simulink model "MPC_3Phase_Inverter"  (R2021a)
settings: Solver=ode45  StartTime=0  StopTime=0.5  MaxStep=3.3E-5  RelTol=1e-3  EnableMultiTasking=on
values from neighbouring files (symbols this model uses):
  Cfilter = 40e-6    (= 4e-05)    [init_inverter.m]
  Lfilter = 2.4e-3    (= 0.0024)    [init_inverter.m]
  Res = 50    [init_inverter.m]
  Ts = 1e-5    (= 1e-05)    [init_inverter.m]
  Vdc = 400    [init_inverter.m]
  Vref = 188    [init_inverter.m]
undefined symbols (not defined in the file or in its folder): i
libraries: simulink x7, spsIGBTDiodeLib x6, spsGroundLib x4, spsThreePhaseSeriesRLCBranchLib x3, spsCurrentMeasurementLib x3, spsThreePhaseVIMeasurementLib x2, spspowerguiLib x2, spsDCVoltageSourceLib x1
settings Model: Creator=ENG.Ihab  LastModifiedBy=Kuhan
settings SolverCC: AlgebraicLoopSolver=TrustRegion  AutoInsertRateTranBlk=on
settings DataIOCC: LimitDataPoints=on  SaveFormat=Array  SignalLoggingSaveFormat=ModelDataLogs  ReturnWorkspaceOutputs=off
settings OptimizationCC: ExpressionDepthLimit=2147483647  LifeSpan=inf
settings DebuggingCC: AlgebraicLoopMsg=none  UnderspecifiedInitializationDetection=Classic  MergeDetectMultiDrivingBlocksExec=none  FcnCallInpInsideContextMsg=warning  UnconnectedInputMsg=none  UnconnectedOutputMsg=none  UnconnectedLineMsg=none  StateNameClashWarn=warning  SFUnexpectedBacktrackingDiag=warning  SFNoUnconditionalDefaultTransitionDiag=warning  SFExecutionAtInitializationDiag=none  SFMachineParentedDataDiag=warning  ArithmeticOperatorsInVariantConditions=warning
settings HardwareCC: ProdBitPerPointer=32  ProdBitPerSizeT=32  ProdBitPerPtrDiffT=32  ProdLargestAtomicFloat=None  ProdIntDivRoundTo=Undefined  ProdEndianess=Unspecified  ProdWordSize=32  ProdHWDeviceType=32-bit Generic
settings ModelReferenceCC: PropagateSignalLabelsOutOfModel=off
settings SFSimCC: SimUseLocalCustomCode=off  SimParseCustomCode=off  CustomCodeUndefinedFunction=UseInterfaceOnly
settings RTWCC: RTWUseLocalCustomCode=off
settings CodeAppCC: StateflowObjectComments=on
settings GRTTargetCC: TargetLangStandard=C89/C90 (ANSI)  CombineOutputUpdateFcns=off  GRTInterface=on
settings ConfigComp: CovMetricSettings=dw  CovSaveCumulativeToWorkspaceVar=on  CovSaveSingleToWorkspaceVar=on  CovExternalEMLEnable=off

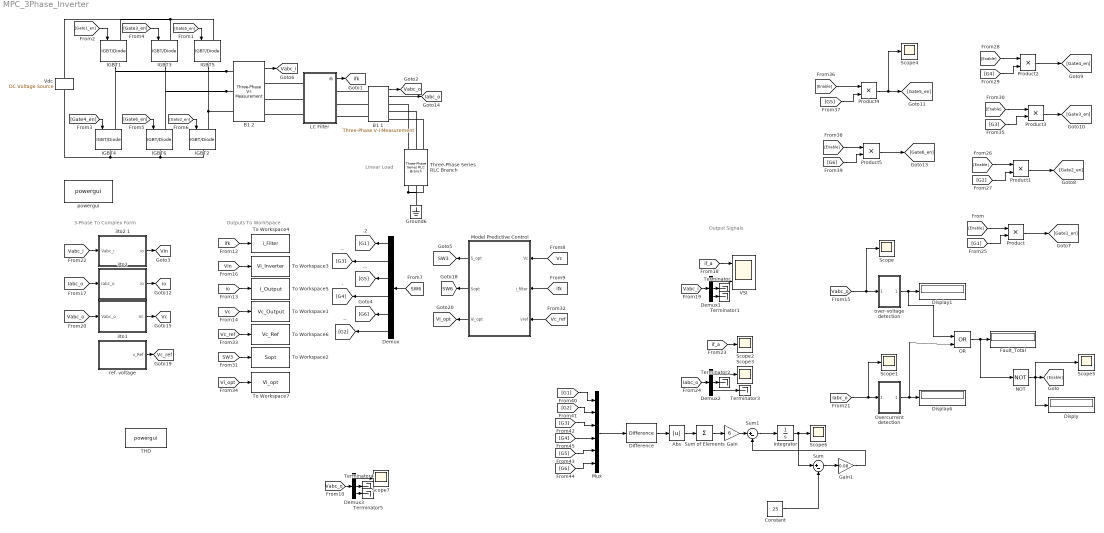
== system MPC_3Phase_Inverter ==
  note: Linear Load
  note: Outputs To WorkSpace
  note: Output Signals
  note: 3-Phase To Complex Form
  3to1 : Subsystem
  "3to2 " : Subsystem
  3to2 1 : Subsystem
  Abs : Abs
  B1 1 : spsThreePhaseVIMeasurementLib/Three-Phase V-I Measurement  VoltageMeasurement=phase-to-ground  SetLabelV=off  LabelV=Vabc  Vpu=off  VpuLL=off  CurrentMeasurement=yes  SetLabelI=off  LabelI=Iabc  Ipu=off  Pbase=100e6  Vbase=500e3  OutputType=Complex  PhasorSimulation=off  PSBequivalent=0
  B1 2 : spsThreePhaseVIMeasurementLib/Three-Phase V-I Measurement  VoltageMeasurement=phase-to-ground  SetLabelV=off  LabelV=Vabc  Vpu=off  VpuLL=off  CurrentMeasurement=no  SetLabelI=off  LabelI=Iabc  Ipu=off  Pbase=100e6  Vbase=500e3  OutputType=Complex  PhasorSimulation=off  PSBequivalent=0
  Constant : Constant  Value=25
  Demux : Demux  Outputs=6
  Demux1 : Demux  Outputs=3
  Demux2 : Demux  Outputs=3
  Demux3 : Demux  Outputs=3
  Difference : simulink/Discrete/Difference  ICPrevInput=0.0  OutMin=[]  OutMax=[]  OutDataType=fixdt(1, 16)  OutScaling=2^-10  DoSatur=off
  Display1 : Display
  Display6 : Display
  Disply : Display
  Fault_Total : Display
  Gain : Gain  Gain=6
  Gain1 : Gain  Gain=0.08
  Ground6 : spsGroundLib/Ground  LConnTagsString=a
  IGBT{1..6} (6 alike) : spsIGBTDiodeLib/IGBT//Diode  Ron=1e-3  Rs=1e5  Cs=inf  Measurements=off
  Integrator : Integrator  InitialCondition=25
  LC Filter : Subsystem
  "Model Predictive Control " : MATLAB Function  TreatAsAtomicUnit=on  mask{Ts=Ts, Cfilter=Cfilter, Lfilter=Lfilter, Vdc=Vdc}
      mask prompts: Ts "Sampling Time"; Cfilter "Filter Capacitor"; Lfilter "Filter Inductance"; Vdc "Input DC Voltage"
  Mux : Mux  Inputs=6
  NOT : Logic  Operator=NOT  IconShape=distinctive  AllPortsSameDT=off  OutDataTypeStr=boolean
  OR : Logic  Operator=OR  IconShape=distinctive  AllPortsSameDT=off  OutDataTypeStr=boolean
  Overcurrent detection : Subsystem
  Product{,1..5} (6 alike) : Product
  Scope{,1..7} (8 alike) : Scope
  Sum : Sum  Inputs=|+-
  Sum of Elements : Sum  Inputs=+
  Sum1 : Sum  Inputs=|+-
  THD : spspowerguiLib/powergui  Priority=1  SimulationMode=Continuous  SampleTime=50e-6  frequency=60  Iterations=50  frequencyindice=60  Pbase=100e6  ErrMax=1e-4  UnitsV=kV  UnitsW=MW  buscounter=0  FunctionMessages=off  echomessages=off  EnableUseOfTLC=off  CurrentSourceSwitches=off  DisableSnubberDevices=off  DisableRonSwitches=off  DisableVfSwitches=off  DisplayEquations=off  AutomaticDiscreteSolvers=off  SolverType=Tustin/Backward Euler (TBE)  Interpol=off  ExternalGateDelay=off  methode=off  Ts=100  x0status=blocks  SPID=on  SwTol=0  HookPort=off  NonlinearTolerance=1e-4  nMaxIteration=100  ContinueOnMaxIteration=off  RestoreLinks=warning  ResistiveCurrentMeasurement=off  Frange=[0:2:500]  Ylog=off  Xlog=on  ShowGrid=off  save=off  variable=ZData  structure=0  ZoomFFT=off  StartTime=0.0  cycles=1  DisplayStyle=1  fundamental=60  FreqAxis=off  MaxFrequency=1000  frequencyindicesteady=1  RmsSteady=1  display=off
  Terminator{,1..5} (6 alike) : Terminator
  Three-Phase Series RLC Branch : spsThreePhaseSeriesRLCBranchLib/Three-Phase Series RLC Branch  LConnTagsString=A|B|C  RConnTagsString=A|B|C  BranchType=R  Resistance=Res  Inductance=0.01  Capacitance=40e-6  Measurements=None
  To Workspace1 : ToWorkspace  VariableName=Vc_Output  SampleTime=-1
  To Workspace2 : ToWorkspace  VariableName=Sopt  SaveFormat=Structure With Time  SampleTime=-1
      settings: Save2DSignal=2-D array (concatenate along first dimension)
  To Workspace3 : ToWorkspace  VariableName=Vi_Inverter  SampleTime=-1
  To Workspace4 : ToWorkspace  VariableName=i_Filter  SampleTime=-1
  To Workspace5 : ToWorkspace  VariableName=i_Output  SampleTime=-1
  To Workspace6 : ToWorkspace  VariableName=Vc_Ref  SampleTime=-1
  To Workspace7 : ToWorkspace  VariableName=Vi_opt  SampleTime=-1
      settings: Save2DSignal=2-D array (concatenate along first dimension)
  VSI : Scope  NumInputPorts=2
  Vdc : spsDCVoltageSourceLib/DC Voltage Source  Description=source block  Amplitude=Vdc  Measurements=None
      settings: AttributesFormatString=\n
  over-voltage detection : Subsystem
  powergui : spspowerguiLib/powergui  SimulationMode=Discrete  SampleTime=Ts  frequency=60  Iterations=50  frequencyindice=0  Pbase=100e6  ErrMax=1e-4  UnitsV=kV  UnitsW=MW  buscounter=0  FunctionMessages=off  echomessages=off  EnableUseOfTLC=off  CurrentSourceSwitches=off  DisableSnubberDevices=off  DisableRonSwitches=off  DisableVfSwitches=off  DisplayEquations=off  AutomaticDiscreteSolvers=off  SolverType=Tustin/Backward Euler (TBE)  Interpol=off  ExternalGateDelay=off  methode=off  Ts=100  x0status=blocks  SPID=off  SwTol=0  HookPort=off  NonlinearTolerance=1e-4  nMaxIteration=100  ContinueOnMaxIteration=off  RestoreLinks=warning  ResistiveCurrentMeasurement=off  Frange=[0:2:500]  Ylog=off  Xlog=on  ShowGrid=off  save=off  variable=ZData  structure=Outputs  ZoomFFT=off  StartTime=0.07  cycles=2  DisplayStyle=1  fundamental=50  FreqAxis=on  MaxFrequency=2000  frequencyindicesteady=1  RmsSteady=2  display=off
  ref. voltage : Subsystem
  tag scope: Iabc_o=global, SW3=global, SW6=global, Vabc_i=global, Vabc_o=global, Vc=global, Vc_ref=global, Vi_opt=global, Vin=global, ifk=global, io=global
  wires:
  LC Filter/1(ifk) -> [ifk]
  [Gate4_en] -> IGBT4/1
  [Gate3_en] -> IGBT3/1
  [Gate6_en] -> IGBT6/1
  [Gate2_en] -> IGBT2/1
  [Gate5_en] -> IGBT5/1
  [Gate1_en] -> IGBT1/1
  Demux/1 -> [G1]
  Demux/2 -> [G3]
  Demux/3 -> [G5]
  Demux/4 -> [G4]
  Demux/5 -> [G6]
  Demux/6 -> [G2]
  "Model Predictive Control "/1(S_opt) -> [SW3]
  [SW6] -> Demux/1
  [Vc] -> "Model Predictive Control "/1(Vc)
  [ifk] -> "Model Predictive Control "/2(i_filter)
  [ifk] -> To Workspace4/1
  [Vin] -> To Workspace3/1
  "3to2 "/1(io) -> [io]
  3to1/1(Vc) -> [Vc]
  [io] -> To Workspace5/1
  [Vc] -> To Workspace1/1
  [SW3] -> To Workspace2/1
  "Model Predictive Control "/2(Sopt) -> [SW6]
  [Vc_ref] -> "Model Predictive Control "/3(vref)
  [Vc_ref] -> To Workspace6/1
  ref. voltage/1(v_Ref) -> [Vc_ref]
  "Model Predictive Control "/3(Vi_opt) -> [Vi_opt]
  [Vi_opt] -> To Workspace7/1
  B1 1/2 -> [Iabc_o]
  [Iabc_o] -> "3to2 "/1("Iabc_o ")
  B1 1/1 -> [Vabc_o]
  [Vabc_o] -> 3to1/1("Vabc_o ")
  B1 2/1 -> [Vabc_i]
  [Vabc_i] -> 3to2 1/1("Vabc_i ")
  3to2 1/1(io) -> [Vin]
  [if_a] -> VSI/1
  Demux1/2 -> Terminator/1
  [Vabc_i] -> Demux1/1
  Demux1/1 -> VSI/2
  Demux1/3 -> Terminator1/1
  [Vabc_o] -> over-voltage detection/1(In1), Scope/1
  [if_a] -> Scope2/1
  Demux2/3 -> Terminator3/1
  [Iabc_o] -> Demux2/1
  Demux2/2 -> Terminator2/1
  Demux2/1 -> Scope3/1
  [Iabc_o] -> Scope1/1, Overcurrent detection/1(In1)
  Overcurrent detection/1(Out1) -> OR/2, Display6/1
  over-voltage detection/1(Out1) -> OR/1, Display1/1
  OR/1 -> NOT/1, Fault_Total/1
  [Enable] -> Product/1
  [G1] -> Product/2
  Product/1 -> [Gate1_en]
  [Enable] -> Product1/1
  [G2] -> Product1/2
  Product1/1 -> [Gate2_en]
  [G4] -> Product2/2
  Product2/1 -> [Gate4_en]
  [Enable] -> Product2/1
  [G3] -> Product3/2
  Product3/1 -> [Gate3_en]
  [Enable] -> Product3/1
  [G5] -> Product4/2
  [Enable] -> Product4/1
  Product4/1 -> Scope4/1, [Gate5_en]
  [G6] -> Product5/2
  [Enable] -> Product5/1
  Product5/1 -> [Gate6_en]
  NOT/1 -> Scope5/1, Disply/1, [Enable]
  Difference/1 -> Abs/1
  [G1] -> Mux/1
  [G2] -> Mux/2
  [G4] -> Mux/4
  [G3] -> Mux/3
  [G5] -> Mux/5
  [G6] -> Mux/6
  Mux/1 -> Difference/1
  Abs/1 -> Sum of Elements/1
  Sum of Elements/1 -> Gain/1
  Integrator/1 -> Sum/1, Scope6/1
  Constant/1 -> Sum/2
  Sum/1 -> Gain1/1
  Gain/1 -> Sum1/1
  Sum1/1 -> Integrator/1
  Gain1/1 -> Sum1/2
  Demux3/3 -> Terminator5/1
  Demux3/1 -> Scope7/1
  [Vabc_o] -> Demux3/1
  Demux3/2 -> Terminator4/1
  connections:
  IGBT2/RConn1 -- IGBT6/RConn1 -- Vdc/LConn1 -- IGBT4/RConn1
  IGBT1/LConn1 -- Vdc/RConn1 -- IGBT3/LConn1 -- IGBT5/LConn1
  B1 2/LConn1 -- IGBT4/LConn1 -- IGBT1/RConn1
  IGBT5/RConn1 -- B1 2/LConn3 -- IGBT2/LConn1
  B1 2/LConn2 -- IGBT6/LConn1 -- IGBT3/RConn1
  B1 1/LConn3 -- LC Filter/RConn3
  B1 1/LConn2 -- LC Filter/RConn2
  B1 1/LConn1 -- LC Filter/RConn1
  Three-Phase Series RLC Branch/RConn1 -- B1 1/RConn1
  Three-Phase Series RLC Branch/RConn2 -- B1 1/RConn2
  Three-Phase Series RLC Branch/RConn3 -- B1 1/RConn3
  LC Filter/LConn3 -- B1 2/RConn3
  LC Filter/LConn2 -- B1 2/RConn2
  LC Filter/LConn1 -- B1 2/RConn1
  Three-Phase Series RLC Branch/LConn1 -- Three-Phase Series RLC Branch/LConn2 -- Three-Phase Series RLC Branch/LConn3 -- Ground6/LConn1

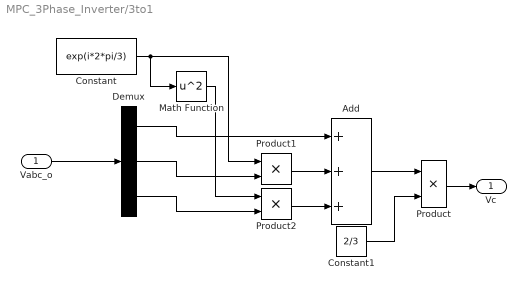
== system MPC_3Phase_Inverter/3to1 ==
  "Vabc_o " : Inport
  Add : Sum  Inputs=+++
  Constant : Constant  Value=exp(i*2*pi/3)
  Constant1 : Constant  Value=2/3
  Demux : Demux  Outputs=3
  Math Function : Math  Operator=square  SignedPower=on  SaturateOnIntegerOverflow=on
  Product : Product  RndMeth=Zero
  Product1 : Product  RndMeth=Zero
  Product2 : Product  RndMeth=Zero
  Vc : Outport  VectorParamsAs1DForOutWhenUnconnected=off
  wires:
  Demux/2 -> Product1/2
  Demux/3 -> Product2/2
  Product2/1 -> Add/3
  Constant1/1 -> Product/2
  Math Function/1 -> Product2/1
  Product/1 -> Vc/1
  Add/1 -> Product/1
  "Vabc_o "/1 -> Demux/1
  Constant/1 -> Product1/1, Math Function/1
  Demux/1 -> Add/1
  Product1/1 -> Add/2

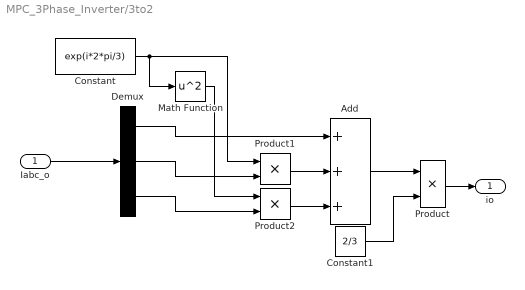
== system MPC_3Phase_Inverter/3to2  ==
  "Iabc_o " : Inport
  Add : Sum  Inputs=+++
  Constant : Constant  Value=exp(i*2*pi/3)
  Constant1 : Constant  Value=2/3
  Demux : Demux  Outputs=3
  Math Function : Math  Operator=square  SignedPower=on  SaturateOnIntegerOverflow=on
  Product : Product  RndMeth=Zero
  Product1 : Product  RndMeth=Zero
  Product2 : Product  RndMeth=Zero
  io : Outport  VectorParamsAs1DForOutWhenUnconnected=off
  wires:
  Add/1 -> Product/1
  Demux/1 -> Add/1
  Constant1/1 -> Product/2
  Product1/1 -> Add/2
  Constant/1 -> Product1/1, Math Function/1
  Demux/2 -> Product1/2
  Math Function/1 -> Product2/1
  Demux/3 -> Product2/2
  Product2/1 -> Add/3
  Product/1 -> io/1
  "Iabc_o "/1 -> Demux/1

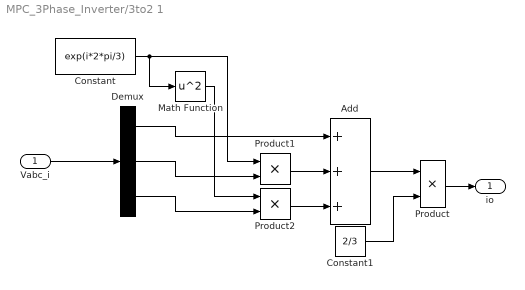
== system MPC_3Phase_Inverter/3to2 1 ==
  "Vabc_i " : Inport
  Add : Sum  Inputs=+++
  Constant : Constant  Value=exp(i*2*pi/3)
  Constant1 : Constant  Value=2/3
  Demux : Demux  Outputs=3
  Math Function : Math  Operator=square  SignedPower=on  SaturateOnIntegerOverflow=on
  Product : Product  RndMeth=Zero
  Product1 : Product  RndMeth=Zero
  Product2 : Product  RndMeth=Zero
  io : Outport  VectorParamsAs1DForOutWhenUnconnected=off
  wires:
  Add/1 -> Product/1
  Demux/1 -> Add/1
  Constant1/1 -> Product/2
  Product1/1 -> Add/2
  Constant/1 -> Product1/1, Math Function/1
  Demux/2 -> Product1/2
  Math Function/1 -> Product2/1
  Demux/3 -> Product2/2
  Product2/1 -> Add/3
  Product/1 -> io/1
  "Vabc_i "/1 -> Demux/1

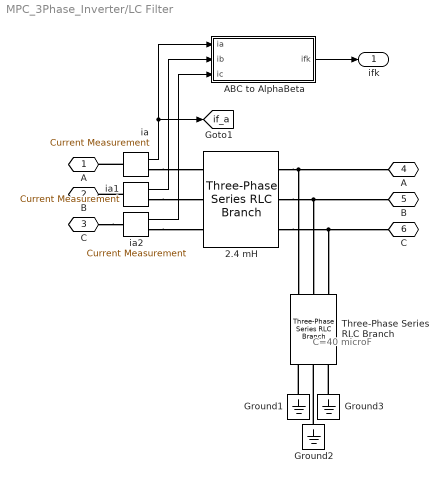
== system MPC_3Phase_Inverter/LC Filter ==
  note: C=40 microF
  "2.4 mH " : spsThreePhaseSeriesRLCBranchLib/Three-Phase Series RLC Branch  LConnTagsString=A|B|C  RConnTagsString=A|B|C  BranchType=L  Resistance=1.0  Inductance=Lfilter  Capacitance=1.0  Measurements=None
  "ABC to AlphaBeta " : Subsystem
  Ground1 : spsGroundLib/Ground  LConnTagsString=a
  Ground2 : spsGroundLib/Ground  LConnTagsString=a
  Ground3 : spsGroundLib/Ground  LConnTagsString=a
  Three-Phase Series RLC Branch : spsThreePhaseSeriesRLCBranchLib/Three-Phase Series RLC Branch  LConnTagsString=A|B|C  RConnTagsString=A|B|C  BranchType=C  Resistance=1  Inductance=1e-3  Capacitance=Cfilter  Measurements=None
  ia : spsCurrentMeasurementLib/Current Measurement  PhasorSimulation=off  OutputType=Complex  PSBequivalent=0
  ia1 : spsCurrentMeasurementLib/Current Measurement  PhasorSimulation=off  OutputType=Complex  PSBequivalent=0
  ia2 : spsCurrentMeasurementLib/Current Measurement  PhasorSimulation=off  OutputType=Complex  PSBequivalent=0
  A : PMIOPort  Side=Left
  B : PMIOPort  Port=2  Side=Left
  C : PMIOPort  Port=3  Side=Left
  "A " : PMIOPort  Port=4  Side=Right
  "B " : PMIOPort  Port=5  Side=Right
  "C " : PMIOPort  Port=6  Side=Right
  ifk : Outport  VectorParamsAs1DForOutWhenUnconnected=off
  tag scope: if_a=global
  wires:
  ia/1 -> [if_a], "ABC to AlphaBeta "/1(ia)
  ia1/1 -> "ABC to AlphaBeta "/2(ib)
  ia2/1 -> "ABC to AlphaBeta "/3(ic)
  "ABC to AlphaBeta "/1(ifk) -> ifk/1
  connections:
  "2.4 mH "/RConn1 -- Three-Phase Series RLC Branch/RConn1 -- "A "/RConn1
  "2.4 mH "/RConn2 -- Three-Phase Series RLC Branch/RConn2 -- "B "/RConn1
  "2.4 mH "/RConn3 -- Three-Phase Series RLC Branch/RConn3 -- "C "/RConn1
  ia/LConn1 -- A/RConn1
  ia/RConn1 -- "2.4 mH "/LConn1
  ia1/LConn1 -- B/RConn1
  C/RConn1 -- ia2/LConn1
  ia1/RConn1 -- "2.4 mH "/LConn2
  ia2/RConn1 -- "2.4 mH "/LConn3
  Ground1/LConn1 -- Three-Phase Series RLC Branch/LConn1
  Ground2/LConn1 -- Three-Phase Series RLC Branch/LConn2
  Ground3/LConn1 -- Three-Phase Series RLC Branch/LConn3

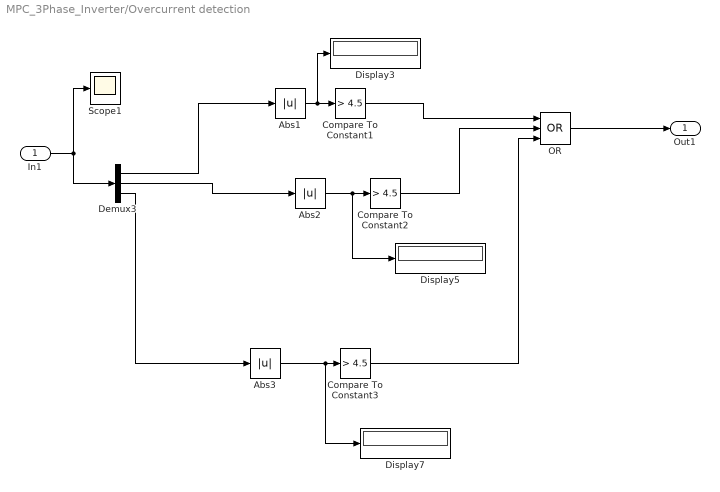
== system MPC_3Phase_Inverter/Overcurrent detection ==
  In1 : Inport
  Abs1 : Abs
  Abs2 : Abs
  Abs3 : Abs
  Compare To Constant1 : simulink/Logic and Bit Operations/Compare To Constant  relop=>  const=4.5  OutDataTypeStr=boolean
  Compare To Constant2 : simulink/Logic and Bit Operations/Compare To Constant  relop=>  const=4.5  OutDataTypeStr=boolean
  Compare To Constant3 : simulink/Logic and Bit Operations/Compare To Constant  relop=>  const=4.5  OutDataTypeStr=boolean
  Demux3 : Demux  Outputs=3
  Display3 : Display
  Display5 : Display
  Display7 : Display
  OR : Logic  Operator=OR  Inputs=3  IconShape=distinctive  AllPortsSameDT=off  OutDataTypeStr=boolean
  Scope1 : Scope
  Out1 : Outport
  wires:
  Abs3/1 -> Display7/1, Compare To Constant3/1
  Demux3/1 -> Abs1/1
  Compare To Constant2/1 -> OR/2
  In1/1 -> Scope1/1, Demux3/1
  Abs1/1 -> Display3/1, Compare To Constant1/1
  Demux3/2 -> Abs2/1
  Compare To Constant3/1 -> OR/3
  Abs2/1 -> Display5/1, Compare To Constant2/1
  Compare To Constant1/1 -> OR/1
  Demux3/3 -> Abs3/1
  OR/1 -> Out1/1

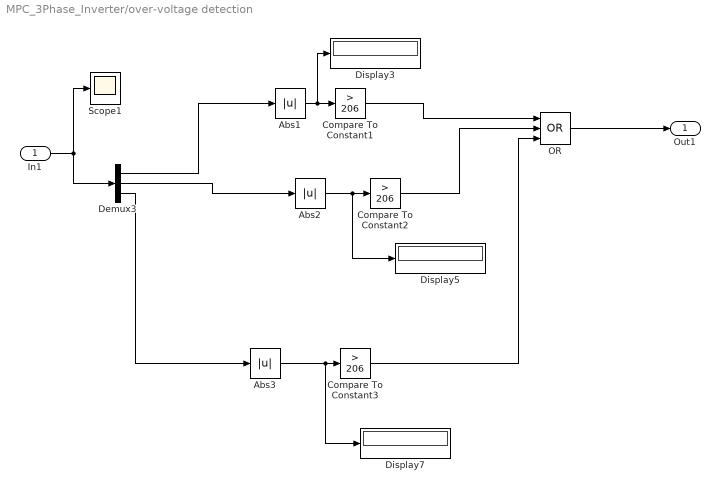
== system MPC_3Phase_Inverter/over-voltage detection ==
  In1 : Inport
  Abs1 : Abs
  Abs2 : Abs
  Abs3 : Abs
  Compare To Constant1 : simulink/Logic and Bit Operations/Compare To Constant  relop=>  const=206  OutDataTypeStr=boolean
  Compare To Constant2 : simulink/Logic and Bit Operations/Compare To Constant  relop=>  const=206  OutDataTypeStr=boolean
  Compare To Constant3 : simulink/Logic and Bit Operations/Compare To Constant  relop=>  const=206  OutDataTypeStr=boolean
  Demux3 : Demux  Outputs=3
  Display3 : Display
  Display5 : Display
  Display7 : Display
  OR : Logic  Operator=OR  Inputs=3  IconShape=distinctive  AllPortsSameDT=off  OutDataTypeStr=boolean
  Scope1 : Scope
  Out1 : Outport
  wires:
  Abs3/1 -> Display7/1, Compare To Constant3/1
  Demux3/1 -> Abs1/1
  Compare To Constant2/1 -> OR/2
  In1/1 -> Scope1/1, Demux3/1
  Abs1/1 -> Display3/1, Compare To Constant1/1
  Demux3/2 -> Abs2/1
  Compare To Constant3/1 -> OR/3
  Abs2/1 -> Display5/1, Compare To Constant2/1
  Compare To Constant1/1 -> OR/1
  Demux3/3 -> Abs3/1
  OR/1 -> Out1/1

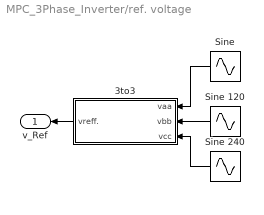
== system MPC_3Phase_Inverter/ref. voltage ==
  3to3 : Subsystem
  Sine : Sin  Amplitude=Vref  Frequency=100*pi  SampleTime=Ts
  Sine 120 : Sin  Amplitude=Vref  Frequency=100*pi  Phase=(2*pi)/3  SampleTime=Ts
  Sine 240 : Sin  Amplitude=Vref  Frequency=100*pi  Phase=(4*pi)/3  SampleTime=Ts
  v_Ref : Outport  VectorParamsAs1DForOutWhenUnconnected=off
  wires:
  Sine/1 -> 3to3/1(vaa)
  Sine 120/1 -> 3to3/2(vbb)
  Sine 240/1 -> 3to3/3(vcc)
  3to3/1(vreff.) -> v_Ref/1

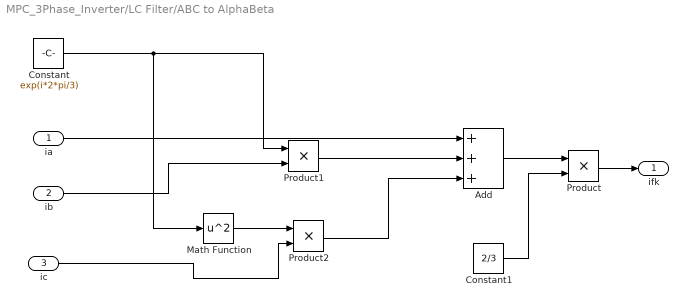
== system MPC_3Phase_Inverter/LC Filter/ABC to AlphaBeta  ==
  ia : Inport
  ib : Inport  Port=2
  ic : Inport  Port=3
  Add : Sum  Inputs=+++
  Constant : Constant  Value=exp(i*2*pi/3)
  Constant1 : Constant  Value=2/3
  Math Function : Math  Operator=square  SignedPower=on  SaturateOnIntegerOverflow=on
  Product : Product  RndMeth=Zero
  Product1 : Product  RndMeth=Zero
  Product2 : Product  RndMeth=Zero
  ifk : Outport  VectorParamsAs1DForOutWhenUnconnected=off
  wires:
  Add/1 -> Product/1
  ia/1 -> Add/1
  Constant1/1 -> Product/2
  Product1/1 -> Add/2
  Constant/1 -> Product1/1, Math Function/1
  ib/1 -> Product1/2
  Math Function/1 -> Product2/1
  ic/1 -> Product2/2
  Product2/1 -> Add/3
  Product/1 -> ifk/1

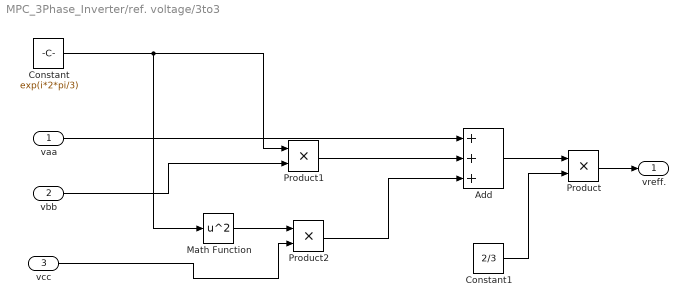
== system MPC_3Phase_Inverter/ref. voltage/3to3 ==
  vaa : Inport
  vbb : Inport  Port=2
  vcc : Inport  Port=3
  Add : Sum  Inputs=+++
  Constant : Constant  Value=exp(i*2*pi/3)
  Constant1 : Constant  Value=2/3
  Math Function : Math  Operator=square  SignedPower=on  SaturateOnIntegerOverflow=on
  Product : Product  RndMeth=Zero
  Product1 : Product  RndMeth=Zero
  Product2 : Product  RndMeth=Zero
  vreff. : Outport  VectorParamsAs1DForOutWhenUnconnected=off
  wires:
  Add/1 -> Product/1
  vaa/1 -> Add/1
  Constant1/1 -> Product/2
  Product1/1 -> Add/2
  Constant/1 -> Product1/1, Math Function/1
  vbb/1 -> Product1/2
  Math Function/1 -> Product2/1
  vcc/1 -> Product2/2
  Product2/1 -> Add/3
  Product/1 -> vreff./1

== matlab function MPC_3Phase_Inverter/Model Predictive Control  ==
  settings: sampleTime=33*1e-6
  data: S_opt output; Sopt output; Vc input; i_filter input; vref input; Vi_opt output; Vdc parameter double size=1; Ts parameter size=1; Cfilter parameter size=1; Lfilter parameter size=1
function [S_opt, Sopt, Vi_opt] = MPC(Vc,i_filter,vref,Vdc,Ts,Cfilter,Lfilter)

    % In order to call "cont2dis" function
    coder.extrinsic('cont2dis');
    persistent Aq Bq Bdq Vc1 Vc_old if_old x_opt g 

    % Initialize variables and get the parameters of the Discrete model based on Ts
    if isempty(x_opt), x_opt = 1; end
    if isempty(Vc1), Vc1 = 0 + 1j*0; end
    if isempty(Vc_old), Vc_old = 0 + 1j*0; end
    if isempty(if_old), if_old = 0 + 1j*0; end
    
    if isempty(Aq) && isempty(Bq) && isempty(Bdq)
        Aq = zeros(2);     Bq = zeros(2,1);     Bdq = zeros(2,1);
        % Call "cont2dis" function
        [Aq, Bq, Bdq] = cont2dis(Ts,Lfilter,Cfilter); 
    end
    
    % Intialize the cost function
    g_opt = inf;
    
    % To generate the switching states matrix
    states = [1 0 0;
              1 1 0
              0 1 0
              0 1 1
              0 0 1
              1 0 1
              1 1 1];
    a = exp(1j*(2*pi/3));
    
    % Read current measurements at sampling instant k
    ifk = i_filter;
    Vck = Vc;
    % Equation of io(k-1) = if(k-1)-(c/Ts)(vc(k)-vc(k-1)).
    io = if_old - (Cfilter/Ts)*(Vck - Vc_old); 
    
    % Store the measured current for the next iteration
    if_old = ifk;
    Vc_old = Vck;
    % FOR loop to find the best switch in the next instant and its corresponding V(i)
    for k = 1:7
        s = states(k,:);
        sw = (2/3)*(s(1)+a*s(2)+a^2*s(3));
        Vi = Vdc*sw;

        % Output Voltage Prediction at instant k+1
        Vc1 = Aq(2,1)*ifk + Aq(2,2)*Vck + Bq(2)*Vi + Bdq(2)*io; 
                
        g = (real(vref)-real(Vc1))^2+(imag(vref)-imag(Vc1))^2;
        if (g < g_opt)
            x_opt = k;
            g_opt = g;
        end  
    end
    % Output switching states and its voltage vector. 
    Vi_opt = x_opt; 
    S_opt = states(x_opt,:);
    d_opt = not(S_opt);
    Sopt = [S_opt,d_opt];     
end
